simulink model "Hardware_proj3"  (R2021a)
settings: Solver=VariableStepAuto  StartTime=0.0  StopTime=35  RelTol=1e-3
undefined symbols (not defined in the file or in its folder): A, N
libraries: hdlBasic x32, xbsIndex_r4 x1, JTAGRuntimeCosim_r4 x1
settings Model: Creator=jag33  LastModifiedBy=JAG33

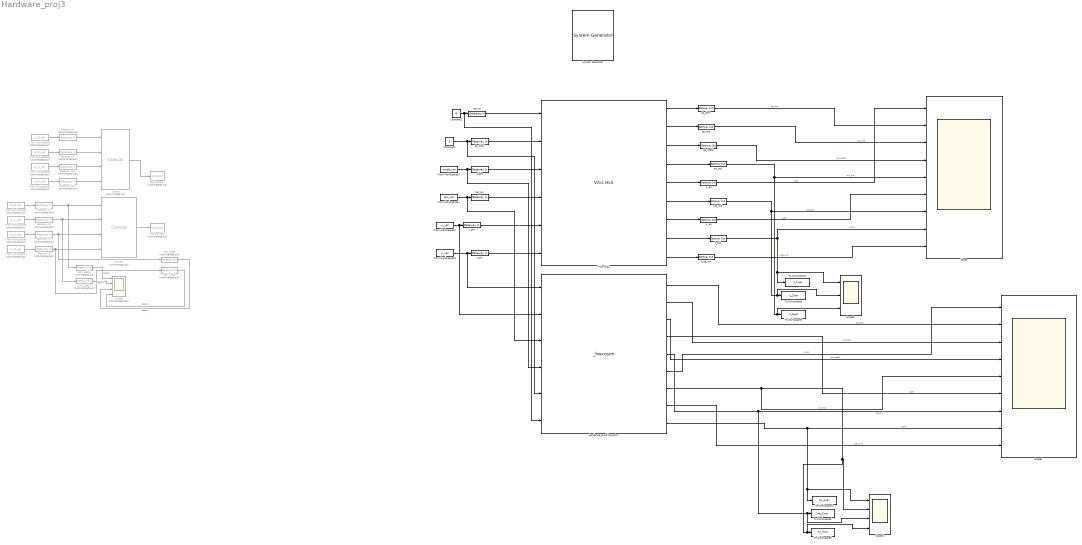
== system Hardware_proj3 ==
  " System Generator" : xbsIndex_r4/ System Generator  Tag=genX  xilinxfamily=zynq  part=xc7z020  speed=-1  package=clg484  synthesis_tool=Vivado  clock_wrapper=Clock Enables  directory=./netlist_proj3  proj_type=Vivado  Synth_file=Vivado Synthesis Defaults  Impl_file=Vivado Implementation Defaults  testbench=off  simulink_period=1  sysclk_period=10  dcm_input_clock_period=10  incr_netlist=off  trim_vbits=Everywhere in SubSystem  dbl_ovrd=According to Block Masks  core_generation=According to Block Masks  run_coregen=off  deprecated_control=off  eval_field=0  block_type=sysgen
  Concat : hdlBasic/Concat  Commented=on  num_inputs=4  XmcBlockStatus=1  maskContainerNames=group1  block_type=concat  block_config=sysgen:Concat_config
  Concat1 : hdlBasic/Concat  Commented=on  num_inputs=4  XmcBlockStatus=1  maskContainerNames=group1  block_type=concat  block_config=sysgen:Concat_config
  Constant1 : Constant
  Constant2 : Constant  Value=0
  From Workspace11 : FromWorkspace  VariableName=tan_var
  From Workspace12 : FromWorkspace  VariableName=x_var
  From Workspace13 : FromWorkspace  VariableName=y_var
  From Workspace14 : FromWorkspace  VariableName=mode_var
  From Workspace2 : FromWorkspace  Commented=on  VariableName=a_i0_var
  From Workspace3 : FromWorkspace  Commented=on  VariableName=a_i1_var
  From Workspace4 : FromWorkspace  Commented=on  VariableName=b_i0_var
  From Workspace5 : FromWorkspace  Commented=on  VariableName=b_i1_var
  From Workspace6 : FromWorkspace  Commented=on  VariableName=b_i2_var
  From Workspace7 : FromWorkspace  Commented=on  VariableName=b_i3_var
  From Workspace8 : FromWorkspace  Commented=on  VariableName=a_i2_var
  From Workspace9 : FromWorkspace  Commented=on  VariableName=a_i3_var
  Gateway In{,1..2,5..7,10..11} (8 alike) : hdlBasic/Gateway In  Commented=on  gui_display_data_type=Fixed-point  arith_type=Unsigned  n_bits=16  bin_pt=0  preci_type=Single  exp_width=8  frac_width=24  rows=1  columns=1  quantization="Round  (unbiased: +/- Inf)"  overflow=Saturate  period=1  UseAsADC=off  ADCChannel='1'  interface=None  automatic_assignment=on  address_offset=hex2dec('00')  intf_name=''  intf_description=''  default_value=0  timing_constraint=None  locs_specified=off  LOCs={}  io_standard={}  inherit_from_input=off  hdl_port=on  XmcBlockStatus=1  maskContainerNames=group4  block_type=gatewayin  block_config=sysgen:gateway_in_config  block_width_w=590  block_height_w=620  block_width=640  block_height=850
  Hardware_proj3 hwcosim : JTAGRuntimeCosim_r4/_hwcosim  clkSrc=Single Stepped  hasCombinationalPath=on  bitfileName=C:\ELEC522\jag33\proj3\netlist_proj3\hardware_proj3.bit  skipConfig=off  dispPartInfo=off  useZynqReconfigScript=on  cable=Auto Detect  speed=N/A  cablePort=N/A  cableLocation=Local  shareCable=off  xmp=[]  software_settings=[]  design_xtable=|  binDir=[]  engineDll=JTAGCosimEngine.dll  cableWaitTime=10  bscanPos=-1  IRLengths=[]  useWaitBox=1  hasBufgmux=on  Scheme=Cosim  useCmdProc=1  hasProc=0  useImpact=0  printLogFile=0  userChain=2  XmcBlockStatus=0  maskContainerNames=tabcontainer1  block_type=jtagcosim  block_config=Sysgen:hwcosim_block_config
      | {
      |     'clkWrapper' => 'hardware_proj3',
      |     'burstMode' => false,
      |     'burstFifoDepth' => '1024',
      |     'shared_memories' => {},
      |     'clocksGcd' => 1,
      |     'device' => {
      |       'family' => 'zynq',
      |       'part' => 'xc7z020',
      |       'package' => 'clg484',
      |       'speed' => '-1',
      |     },
      |     'ports' => {
      |       'y_gin' => {
      |         'direction' => 'in',
      |         'width' => 16,
      |         'name' => 'y_gin',
      |         'period' => 1,
      |         'icon_text' => 'y_gin',
      |         'type' => 'Fix_16_13',
      |         'arithmetic_type' => 'xlSigned',
      |         'dat_file' => 'hardware_proj3_y_gin.dat',
      |         'bin_pt' => 13,
      |         'addr_offset' => 0,
      |         'bd_port_index' => 0,
      |       },
      |       'x_gin' => {
      |         'direction' => 'in',
      |         'width' => 16,
      |         'name' => 'x_gin',
      |         'period' => 1,
      |         'icon_text' => 'x_gin',
      |         'type' => 'Fix_16_13',
      |         'arithmetic_type' => 'xlSigned',
      |         'dat_file' => 'hardware_proj3_x_gin.dat',
      |         'bin_pt' => 13,
      |         'addr_offset' => 4,
      |         'bd_port_index' => 1,
      |       },
      |       'tan_gin' => {
      |         'direction' => 'in',
      |         'width' => 16,
      |         'name' => 'tan_gin',
      |         'period' => 1,
      |         'icon_text' => 'tan_gin',
      |         'type' => 'Fix_16_13',
      |         'arithmetic_type' => 'xlSigned',
      |         'dat_file' => 'hardware_proj3_tan_gin.dat',
      |         'bin_pt' => 13,
      |         'addr_offset' => 8,
      |         'bd_port_index' => 2,
      |       },
      |       'state' => {
      |         'direction' => 'in',
      |         'width' => 1,
      |         'name' => 'state',
      |         'period' => 1,
      |         'icon_text' => 'state',
      |         'type' => 'Bool',
      |         'arithmetic_type' => 'xlUnsigned',
      |         'dat_file' => 'hardware_proj3_state.dat',
      |         'bin_pt' => 0,
      |         'addr_offset' => 12,
      |         'bd_port_index' => 3,
      |       },
      |       'ap_start' => {
      |         'direction' => 'in',
      |         'width' => 1,
      |         'name' => 'ap_start',
      |         'period' => 1,
      |         'icon_text' => 'ap_start',
      |         'type' => 'Bool',
      |         'arithmetic_type' => 'xlUnsigned',
      |         'dat_file' => 'hardware_proj3_ap_start.dat',
      |         'bin_pt' => 0,
      |         'addr_offset' => 16,
      |         'bd_port_index' => 4,
      |       },
      |       'ap_rst' => {
      |         'direction' => 'in',
      |         'width' => 1,
      |         'name' => 'ap_rst',
      |         'period' => 1,
      |         'icon_text' => 'ap_rst',
      |         'type' => 'Bool',
      |         'arithmetic_type' => 'xlUnsigned',
      |         'dat_file' => 'hardware_proj3_ap_rst.dat',
      |         'bin_pt' => 0,
      |         'addr_offset' => 20,
      |         'bd_port_index' => 5,
      |       },
      |       'ap_donr' => {
      |         'direction' => 'out',
      |         'width' => 1,
      |         'name' => 'ap_donr',
      |         'period' => 1,
      |         'icon_text' => 'ap_donr',
      |         'type' => 'Bool',
      |         'arithmetic_type' => 'xlUnsigned',
      |         'dat_file' => 'hardware_proj3_ap_donr.dat',
      |         'bin_pt' => 0,
      |         'addr_offset' => 24,
      |         'bd_port_index' => 0,
      |       },
      |       'ap_idle' => {
      |         'direction' => 'out',
      |         'width' => 1,
      |         'name' => 'ap_idle',
      |         'period' => 1,
      |         'icon_text' => 'ap_idle',
      |         'type' => 'Bool',
      |         'arithmetic_type' => 'xlUnsigned',
      |         'dat_file' => 'hardware_proj3_ap_idle.dat',
      |         'bin_pt' => 0,
      |         'addr_offset' => 28,
      |         'bd_port_index' => 1,
      |       },
      |       'ap_ready' => {
      |         'direction' => 'out',
      |         'width' => 1,
      |         'name' => 'ap_ready',
      |         'period' => 1,
      |         'icon_text' => 'ap_ready',
      |         'type' => 'Bool',
      |         'arithmetic_type' => 'xlUnsigned',
      |         'dat_file' => 'hardware_proj3_ap_ready.dat',
      |         'bin_pt' => 0,
      |         'addr_offset' => 32,
      |         'bd_port_index' => 2,
      |       },
      |       'c_ap' => {
      |         'direction' => 'out',
      |         'width' => 1,
      |         'name' => 'c_ap',
      |         'period' => 1,
      |         'icon_text' => 'c_ap',
      |         'type' => 'Bool',
      |         'arithmetic_type' => 'xlUnsigned',
      |         'dat_file' => 'hardware_proj3_c_ap.dat',
      |         'bin_pt' => 0,
      |         'addr_offset' => 36,
      |         'bd_port_index' => 3,
      |       },
      |       'cos_out' => {
      |         'direction' => 'out',
      |         'width' => 16,
      |         'name' => 'cos_out',
      |         'period' => 1,
      |         'icon_text' => 'cos_out',
      |         'type' => 'Fix_16_13',
      |         'arithmetic_type' => 'xlSigned',
      |         'dat_file' => 'hardware_proj3_cos_out.dat',
      |         'bin_pt' => 13,
      |         'addr_offset' => 40,
      |         'bd_port_index' => 4,
      |       },
      |       's_ap' => {
      |         'direction' => 'out',
      |         'width' => 1,
      |         'name' => 's_ap',
      |         'period' => 1,
      |         'icon_text' => 's_ap',
      |         'type' => 'Bool',
      |         'arithmetic_type' => 'xlUnsigned',
      |         'dat_file' => 'hardware_proj3_s_ap.dat',
      |         'bin_pt' => 0,
      |         'addr_offset' => 44,
      |         'bd_port_index' => 5,
      |       },
      |       'sin_out' => {
      |         'direction' => 'out',
      |         'width' => 16,
      |         'name' => 'sin_out',
      |         'period' => 1,
      |         'icon_text' => 'sin_out',
      |         'type' => 'Fix_16_13',
      |         'arithmetic_type' => 'xlSigned',
      |         'dat_file' => 'hardware_proj3_sin_out.dat',
      |         'bin_pt' => 13,
      |         'addr_offset' => 48,
      |         'bd_port_index' => 6,
      |       },
      |       't_ap_vld' => {
      |         'direction' => 'out',
      |         'width' => 1,
      |         'name' => 't_ap_vld',
      |         'period' => 1,
      |         'icon_text' => 't_ap_vld',
      |         'type' => 'Bool',
      |         'arithmetic_type' => 'xlUnsigned',
      |         'dat_file' => 'hardware_proj3_t_ap_vld.dat',
      |         'bin_pt' => 0,
      |         'addr_offset' => 52,
      |         'bd_port_index' => 7,
      |       },
      |       't_out' => {
      |         'direction' => 'out',
      |         'width' => 16,
      |         'name' => 't_out',
      |         'period' => 1,
      |         'icon_text' => 't_out',
      |         'type' => 'Fix_16_13',
      |         'arithmetic_type' => 'xlSigned',
      |         'dat_file' => 'hardware_proj3_t_out.dat',
      |         'bin_pt' => 13,
      |         'addr_offset' => 56,
      |         'bd_port_index' => 8,
      |       },
      |     },
      |   }
  Reinterpret : hdlBasic/Reinterpret  Commented=on  force_arith_type=on  arith_type="Signed  (2's comp)"  force_bin_pt=off  bin_pt=0  XmcBlockStatus=1  maskContainerNames=group1  block_type=reinterpret  block_config=sysgen:Reinterpret_config
  Reinterpret1 : hdlBasic/Reinterpret  Commented=on  force_arith_type=on  arith_type="Signed  (2's comp)"  force_bin_pt=off  bin_pt=0  XmcBlockStatus=1  maskContainerNames=group1  block_type=reinterpret  block_config=sysgen:Reinterpret_config
  Scope : Scope  NumInputPorts=9
  Scope1 : Scope  NumInputPorts=9
  Scope2 : Scope  Commented=on  NumInputPorts=4
  Scope3 : Scope  NumInputPorts=3
  Scope4 : Scope  NumInputPorts=4
  To Workspace1 : ToWorkspace  VariableName=c_1var  SaveFormat=Timeseries  SampleTime=-1
  To Workspace2 : ToWorkspace  VariableName=c_2var  SaveFormat=Timeseries  SampleTime=-1
  To Workspace3 : ToWorkspace  VariableName=c_3var  SaveFormat=Timeseries  SampleTime=-1
  To Workspace4 : ToWorkspace  VariableName=hc_1var  SaveFormat=Timeseries  SampleTime=-1
  To Workspace5 : ToWorkspace  VariableName=hc_2var  SaveFormat=Timeseries  SampleTime=-1
  To Workspace6 : ToWorkspace  VariableName=hc_3var  SaveFormat=Timeseries  SampleTime=-1
  Vitis HLS1 : hdlBasic/Vitis HLS  anytable='.\cordic\solution1'  fast_sim=off  display_datatype=on  rate_propagation_method=Simulink system period  model_file_path=''  latency=1  block_type=vitis_hls
      settings: infoedit=This block allows including C,C++ and SystemC source files in System Generator for DSP designs.
  ap_donr : hdlBasic/Gateway Out  inherit_from_input=off  hdl_port=on  rows=1  columns=1  UseAsDAC=off  DACChannel='1'  interface=None  automatic_assignment=on  address_offset=hex2dec('00')  intf_name=''  intf_description=''  timing_constraint=None  locs_specified=off  LOCs={}  io_standard={}  XmcBlockStatus=1  maskContainerNames=group4  block_type=gatewayout  block_config=sysgen:gateway_out_config  block_width_w=590  block_height_w=620  block_width=620  block_height=750
  ap_idle : hdlBasic/Gateway Out  inherit_from_input=off  hdl_port=on  rows=1  columns=1  UseAsDAC=off  DACChannel='1'  interface=None  automatic_assignment=on  address_offset=hex2dec('00')  intf_name=''  intf_description=''  timing_constraint=None  locs_specified=off  LOCs={}  io_standard={}  XmcBlockStatus=1  maskContainerNames=group4  block_type=gatewayout  block_config=sysgen:gateway_out_config  block_width_w=590  block_height_w=620  block_width=620  block_height=750
  ap_ready : hdlBasic/Gateway Out  inherit_from_input=off  hdl_port=on  rows=1  columns=1  UseAsDAC=off  DACChannel='1'  interface=None  automatic_assignment=on  address_offset=hex2dec('00')  intf_name=''  intf_description=''  timing_constraint=None  locs_specified=off  LOCs={}  io_standard={}  XmcBlockStatus=1  maskContainerNames=group4  block_type=gatewayout  block_config=sysgen:gateway_out_config  block_width_w=590  block_height_w=620  block_width=620  block_height=750
  ap_rst : hdlBasic/Gateway In  gui_display_data_type=Boolean  arith_type=Boolean  n_bits=16  bin_pt=0  preci_type=Single  exp_width=8  frac_width=24  rows=1  columns=1  quantization="Round  (unbiased: +/- Inf)"  overflow=Saturate  period=1  UseAsADC=off  ADCChannel='1'  interface=None  automatic_assignment=on  address_offset=hex2dec('00')  intf_name=''  intf_description=''  default_value=0  timing_constraint=None  locs_specified=off  LOCs={}  io_standard={}  inherit_from_input=off  hdl_port=on  XmcBlockStatus=1  maskContainerNames=group4  block_type=gatewayin  block_config=sysgen:gateway_in_config  block_width_w=590  block_height_w=620  block_width=640  block_height=850
  ap_start : hdlBasic/Gateway In  gui_display_data_type=Boolean  arith_type=Boolean  n_bits=16  bin_pt=14  preci_type=Single  exp_width=8  frac_width=24  rows=1  columns=1  quantization="Round  (unbiased: +/- Inf)"  overflow=Saturate  period=1  UseAsADC=off  ADCChannel='1'  interface=None  automatic_assignment=on  address_offset=hex2dec('00')  intf_name=''  intf_description=''  default_value=0  timing_constraint=None  locs_specified=off  LOCs={}  io_standard={}  inherit_from_input=off  hdl_port=on  XmcBlockStatus=1  maskContainerNames=group4  block_type=gatewayin  block_config=sysgen:gateway_in_config  block_width_w=590  block_height_w=620  block_width=640  block_height=850
  c_ap : hdlBasic/Gateway Out  inherit_from_input=off  hdl_port=on  rows=1  columns=1  UseAsDAC=off  DACChannel='1'  interface=None  automatic_assignment=on  address_offset=hex2dec('00')  intf_name=''  intf_description=''  timing_constraint=None  locs_specified=off  LOCs={}  io_standard={}  XmcBlockStatus=1  maskContainerNames=group4  block_type=gatewayout  block_config=sysgen:gateway_out_config  block_width_w=590  block_height_w=620  block_width=620  block_height=750
  cos_out : hdlBasic/Gateway Out  inherit_from_input=off  hdl_port=on  rows=1  columns=1  UseAsDAC=off  DACChannel='1'  interface=None  automatic_assignment=on  address_offset=hex2dec('00')  intf_name=''  intf_description=''  timing_constraint=None  locs_specified=off  LOCs={}  io_standard={}  XmcBlockStatus=1  maskContainerNames=group4  block_type=gatewayout  block_config=sysgen:gateway_out_config  block_width_w=590  block_height_w=620  block_width=620  block_height=750
  post_add{8..11} (4 alike) : hdlBasic/Gateway Out  Commented=on  inherit_from_input=on  hdl_port=on  rows=1  columns=1  UseAsDAC=off  DACChannel='1'  interface=None  automatic_assignment=on  address_offset=hex2dec('00')  intf_name=''  intf_description=''  timing_constraint=None  locs_specified=off  LOCs={}  io_standard={}  XmcBlockStatus=1  maskContainerNames=group4  block_type=gatewayout  block_config=sysgen:gateway_out_config  block_width_w=590  block_height_w=620  block_width=620  block_height=750
  s_ap : hdlBasic/Gateway Out  inherit_from_input=off  hdl_port=on  rows=1  columns=1  UseAsDAC=off  DACChannel='1'  interface=None  automatic_assignment=on  address_offset=hex2dec('00')  intf_name=''  intf_description=''  timing_constraint=None  locs_specified=off  LOCs={}  io_standard={}  XmcBlockStatus=1  maskContainerNames=group4  block_type=gatewayout  block_config=sysgen:gateway_out_config  block_width_w=590  block_height_w=620  block_width=620  block_height=750
  sin_out : hdlBasic/Gateway Out  inherit_from_input=off  hdl_port=on  rows=1  columns=1  UseAsDAC=off  DACChannel='1'  interface=None  automatic_assignment=on  address_offset=hex2dec('00')  intf_name=''  intf_description=''  timing_constraint=None  locs_specified=off  LOCs={}  io_standard={}  XmcBlockStatus=1  maskContainerNames=group4  block_type=gatewayout  block_config=sysgen:gateway_out_config  block_width_w=590  block_height_w=620  block_width=620  block_height=750
  state : hdlBasic/Gateway In  gui_display_data_type=Boolean  arith_type=Boolean  n_bits=16  bin_pt=14  preci_type=Single  exp_width=8  frac_width=24  rows=1  columns=1  quantization="Round  (unbiased: +/- Inf)"  overflow=Saturate  period=1  UseAsADC=off  ADCChannel='1'  interface=None  automatic_assignment=on  address_offset=hex2dec('00')  intf_name=''  intf_description=''  default_value=0  timing_constraint=None  locs_specified=off  LOCs={}  io_standard={}  inherit_from_input=off  hdl_port=on  XmcBlockStatus=1  maskContainerNames=group4  block_type=gatewayin  block_config=sysgen:gateway_in_config  block_width_w=590  block_height_w=620  block_width=640  block_height=850
  t_ap_vld : hdlBasic/Gateway Out  inherit_from_input=off  hdl_port=on  rows=1  columns=1  UseAsDAC=off  DACChannel='1'  interface=None  automatic_assignment=on  address_offset=hex2dec('00')  intf_name=''  intf_description=''  timing_constraint=None  locs_specified=off  LOCs={}  io_standard={}  XmcBlockStatus=1  maskContainerNames=group4  block_type=gatewayout  block_config=sysgen:gateway_out_config  block_width_w=590  block_height_w=620  block_width=620  block_height=750
  t_out : hdlBasic/Gateway Out  inherit_from_input=off  hdl_port=on  rows=1  columns=1  UseAsDAC=off  DACChannel='1'  interface=None  automatic_assignment=on  address_offset=hex2dec('00')  intf_name=''  intf_description=''  timing_constraint=None  locs_specified=off  LOCs={}  io_standard={}  XmcBlockStatus=1  maskContainerNames=group4  block_type=gatewayout  block_config=sysgen:gateway_out_config  block_width_w=590  block_height_w=620  block_width=620  block_height=750
  tan_gin : hdlBasic/Gateway In  gui_display_data_type=Fixed-point  arith_type=Signed (2's comp)  n_bits=16  bin_pt=13  preci_type=Single  exp_width=8  frac_width=24  rows=1  columns=1  quantization="Round  (unbiased: +/- Inf)"  overflow=Saturate  period=1  UseAsADC=off  ADCChannel='1'  interface=None  automatic_assignment=on  address_offset=hex2dec('00')  intf_name=''  intf_description=''  default_value=0  timing_constraint=None  locs_specified=off  LOCs={}  io_standard={}  inherit_from_input=off  hdl_port=on  XmcBlockStatus=1  maskContainerNames=group4  block_type=gatewayin  block_config=sysgen:gateway_in_config  block_width_w=590  block_height_w=620  block_width=640  block_height=850
  x_gin : hdlBasic/Gateway In  gui_display_data_type=Fixed-point  arith_type=Signed (2's comp)  n_bits=16  bin_pt=13  preci_type=Single  exp_width=8  frac_width=24  rows=1  columns=1  quantization="Round  (unbiased: +/- Inf)"  overflow=Saturate  period=1  UseAsADC=off  ADCChannel='1'  interface=None  automatic_assignment=on  address_offset=hex2dec('00')  intf_name=''  intf_description=''  default_value=0  timing_constraint=None  locs_specified=off  LOCs={}  io_standard={}  inherit_from_input=off  hdl_port=on  XmcBlockStatus=1  maskContainerNames=group4  block_type=gatewayin  block_config=sysgen:gateway_in_config  block_width_w=590  block_height_w=620  block_width=640  block_height=850
  y_gin : hdlBasic/Gateway In  gui_display_data_type=Fixed-point  arith_type=Signed (2's comp)  n_bits=16  bin_pt=13  preci_type=Single  exp_width=8  frac_width=24  rows=1  columns=1  quantization="Round  (unbiased: +/- Inf)"  overflow=Saturate  period=1  UseAsADC=off  ADCChannel='1'  interface=None  automatic_assignment=on  address_offset=hex2dec('00')  intf_name=''  intf_description=''  default_value=0  timing_constraint=None  locs_specified=off  LOCs={}  io_standard={}  inherit_from_input=off  hdl_port=on  XmcBlockStatus=1  maskContainerNames=group4  block_type=gatewayin  block_config=sysgen:gateway_in_config  block_width_w=590  block_height_w=620  block_width=640  block_height=850
  wires:
  Vitis HLS1/6 -> cos_out/1
  Vitis HLS1/7 -> c_ap/1
  Vitis HLS1/4 -> sin_out/1
  Vitis HLS1/3 -> ap_ready/1
  Vitis HLS1/2 -> ap_idle/1
  Vitis HLS1/1 -> ap_donr/1
  ap_donr/1 -> Scope/2  "ap_donr"
  ap_idle/1 -> Scope/3  "ap_idle"
  ap_ready/1 -> Scope/4  "ap_ready"
  sin_out/1 -> Scope/5, Scope3/3, To Workspace3/1  "sin_out"
  ap_start/1 -> Vitis HLS1/2
  Vitis HLS1/5 -> s_ap/1
  From Workspace5/1 -> Gateway In5/1
  From Workspace8/1 -> Gateway In10/1
  From Workspace4/1 -> Gateway In2/1
  From Workspace9/1 -> Gateway In11/1
  From Workspace3/1 -> Gateway In1/1
  From Workspace2/1 -> Gateway In/1
  Gateway In2/1 -> post_add11/1, Concat1/1
  Gateway In5/1 -> Concat1/2, post_add10/1
  Gateway In7/1 -> post_add9/1, Concat1/3
  Gateway In6/1 -> post_add8/1, Concat1/4
  Concat1/1 -> Reinterpret1/1
  Gateway In/1 -> Concat/1
  Gateway In1/1 -> Concat/2
  Gateway In10/1 -> Concat/3
  Concat/1 -> Reinterpret/1
  Gateway In11/1 -> Concat/4
  From Workspace6/1 -> Gateway In7/1
  From Workspace7/1 -> Gateway In6/1
  post_add8/1 -> Scope2/4  "accum"
  post_add11/1 -> Scope2/1  "accum"
  post_add10/1 -> Scope2/2  "accum"
  post_add9/1 -> Scope2/3  "accum"
  Constant1/1 -> Hardware_proj3 hwcosim/5, ap_start/1
  t_out/1 -> To Workspace1/1, Scope3/1, Scope/8  "t_out"
  t_ap_vld/1 -> Scope/9  "t_ap_vld"
  Vitis HLS1/8 -> t_out/1
  Vitis HLS1/9 -> t_ap_vld/1
  s_ap/1 -> Scope/1  "s_ap"
  c_ap/1 -> Scope/6  "c_ap"
  cos_out/1 -> Scope/7, Scope3/2, To Workspace2/1  "cos_out"
  ap_rst/1 -> Vitis HLS1/1
  Constant2/1 -> Hardware_proj3 hwcosim/6, ap_rst/1
  tan_gin/1 -> Vitis HLS1/4
  x_gin/1 -> Vitis HLS1/5
  From Workspace11/1 -> Hardware_proj3 hwcosim/3, tan_gin/1
  From Workspace12/1 -> Hardware_proj3 hwcosim/2, x_gin/1
  From Workspace13/1 -> Hardware_proj3 hwcosim/1, y_gin/1
  y_gin/1 -> Vitis HLS1/6
  state/1 -> Vitis HLS1/3
  From Workspace14/1 -> Hardware_proj3 hwcosim/4, state/1
  Hardware_proj3 hwcosim/6 -> Scope1/1  "s_ap"
  Hardware_proj3 hwcosim/8 -> Scope1/9  "t_ap_vld"
  Hardware_proj3 hwcosim/9 -> To Workspace4/1, Scope4/1, Scope1/8  "t_out"
  Hardware_proj3 hwcosim/5 -> Scope4/3, To Workspace5/1, Scope1/7  "cos_out"
  Hardware_proj3 hwcosim/7 -> Scope4/4, To Workspace6/1, Scope4/2, Scope1/5  "sin_out"
  Hardware_proj3 hwcosim/2 -> Scope1/3  "ap_idle"
  Hardware_proj3 hwcosim/4 -> Scope1/6  "c_ap"
  Hardware_proj3 hwcosim/3 -> Scope1/4  "ap_ready"
  Hardware_proj3 hwcosim/1 -> Scope1/2  "ap_donr"
